simulink model "ObservadorDeEstados"  (R2019a)
settings: Solver=VariableStepAuto  StartTime=0.0  StopTime=10  RelTol=1e-3
undefined symbols (not defined in the file): A, B, C
settings Model: Creator=Cliente  LastModifiedBy=Cliente

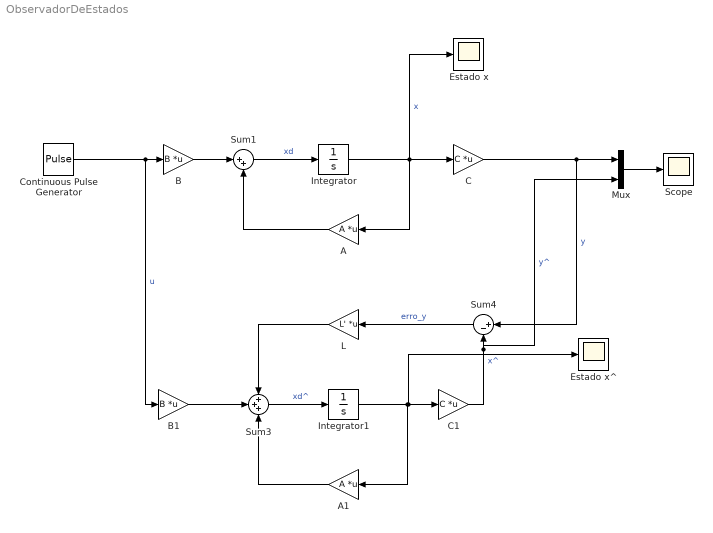
== system ObservadorDeEstados ==
  A : Gain  Gain=A  Multiplication=Matrix(K*u) (u vector)
  A1 : Gain  Gain=A  Multiplication=Matrix(K*u) (u vector)
  B : Gain  Gain=B  Multiplication=Matrix(K*u)
  B1 : Gain  Gain=B  Multiplication=Matrix(K*u)
  C : Gain  Gain=C  Multiplication=Matrix(K*u) (u vector)
  C1 : Gain  Gain=C  Multiplication=Matrix(K*u) (u vector)
  Continuous Pulse Generator : DiscretePulseGenerator  PulseType=Time based  Amplitude=0.1  Period=1  PulseWidth=50
  Estado x : Scope
  Estado x^ : Scope
  Integrator : Integrator  InitialCondition=[0;0]
  Integrator1 : Integrator  InitialCondition=[0;0]
  L : Gain  Gain=L'  Multiplication=Matrix(K*u)
  Mux : Mux  Inputs=2
  Scope : Scope
  Sum1 : Sum  Inputs=|++
  Sum3 : Sum  Inputs=+++
  Sum4 : Sum  Inputs=|+-
  wires:
  C1/1 -> Mux/2, Sum4/2  "y^"
  B1/1 -> Sum3/2
  Sum3/1 -> Integrator1/1  "xd^"
  Integrator/1 -> Estado x/1, C/1, A/1  "x"
  Sum1/1 -> Integrator/1  "xd"
  A1/1 -> Sum3/3
  Sum4/1 -> L/1  "erro_y"
  Integrator1/1 -> A1/1, C1/1, Estado x^/1  "x^"
  L/1 -> Sum3/1
  A/1 -> Sum1/2
  C/1 -> Mux/1, Sum4/1  "y"
  Continuous Pulse Generator/1 -> B1/1, B/1  "u"
  Mux/1 -> Scope/1
  B/1 -> Sum1/1
